simulink model "LOSdemoKF"  (R2016b)
settings: Solver=ode1  StartTime=0.0  StopTime=1200  FixedStep=0.1  RelTol=1e-3
libraries: simulink x1
settings Model: Creator=qys  LastModifiedBy=qys

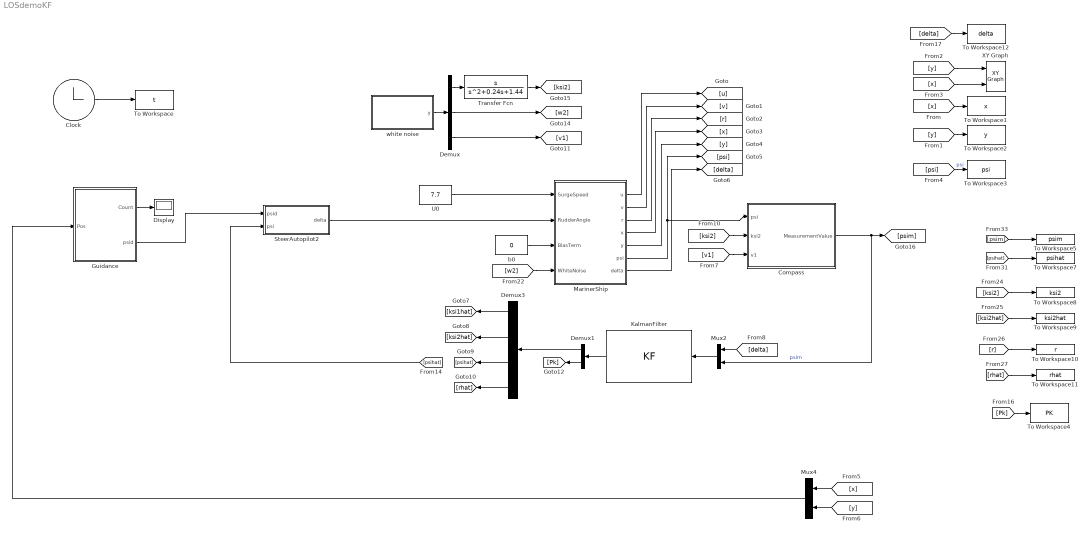
== system LOSdemoKF ==
  Clock : Clock
  Compass : Subsystem
  Demux : Demux  Outputs=3
  Demux1 : Demux  Outputs=[4 16]
  Demux3 : Demux
  Display : Display
  Guidance : Subsystem  mask(Guidance){D=800, R=300, PointSet=[300 300 2900 2500 2900 4800]'}
      mask prompts: D "LookaheadDistance"; R "ChangeRadius"; PointSet "WayPointSet"
      mask help:
      | set lookahead distance\change radius\points number\points set
      | LookaheadDistance: D = 500
      | ChangeRadius: R = 300
      | WayPointSet: PointSet = [0 0 2900 2900 2900 4900 0 0 0 0]'
  KalmanFilter : S-Function  FunctionName=KF  Parameters=Q,R  SFunctionDeploymentMode=off  EnableBusSupport=off  mask(KF4){Q=diag([1e-3 1e-6]), R=1e-2}
      mask prompts: Q "QK"; R "RK"
      mask help:
      | Q = diag([1 1])
      | R = 1
      mask Display: disp('KF4')
  MarinerShip : Subsystem  mask{InitialState=[0;0;0;0;0;0;0]}
      mask Display: disp('mariner1')
  Mux2 : Mux  Inputs=2
  Mux4 : Mux  Inputs=2
  SteerAutopilot2 : Subsystem  mask(PID+TFF){Kp=1.45, Ti=1/100, Td=40}
      mask help:
      | TFF = T*Wxd/K+Wxd/K
      | PID = Kp*[(Xd-X)+Integrate(Xd-X)/Ti+Td*D(Xd-X)]
      | delta = TFF+PID*T/K
      | Kp = T*wn^2/K;
      | Td = T*(2*ksi*wn-1/T)/(K*Kp);
      | Ti = 10/wn;
  To Workspace : ToWorkspace  VariableName=t  SampleTime=-1
  To Workspace1 : ToWorkspace  VariableName=x  SampleTime=-1
  To Workspace10 : ToWorkspace  VariableName=r  SampleTime=-1
  To Workspace11 : ToWorkspace  VariableName=rhat  SampleTime=-1
  To Workspace12 : ToWorkspace  VariableName=delta  SampleTime=-1
  To Workspace2 : ToWorkspace  VariableName=y  SampleTime=-1
  To Workspace3 : ToWorkspace  VariableName=psi  SampleTime=-1
  To Workspace4 : ToWorkspace  VariableName=PK  SampleTime=-1
  To Workspace5 : ToWorkspace  VariableName=psim  SampleTime=-1
  To Workspace7 : ToWorkspace  VariableName=psihat  SampleTime=-1
  To Workspace8 : ToWorkspace  VariableName=ksi2  SampleTime=-1
  To Workspace9 : ToWorkspace  VariableName=ksi2hat  SampleTime=-1
  Transfer Fcn : TransferFcn  Numerator=[1 0]  Denominator=[1 0.24 1.44]
  U0 : Constant  Value=7.7
  XY Graph : simulink/Sinks/XY Graph  xmin=-100  xmax=5000  ymin=-100  ymax=5000  st=-1
  b0 : Constant  Value=0
  white noise : MATLAB Function  TreatAsAtomicUnit=on
  wires:
  U0/1 -> MarinerShip/1(SurgeSpeed)
  Clock/1 -> To Workspace/1
  Mux2/1 -> KalmanFilter/1
  Compass/1(MeasurementValue) -> [psim], Mux2/2  "psim"
  Demux1/1 -> Demux3/1
  Guidance/1(Count) -> Display/1
  Mux4/1 -> Guidance/1(Pos)
  MarinerShip/1(u) -> [u]
  MarinerShip/2(v) -> [v]
  MarinerShip/3(r) -> [r]
  MarinerShip/4(x) -> [x]
  MarinerShip/5(y) -> [y]
  MarinerShip/6(psi) -> [psi], Compass/1(psi)
  MarinerShip/7(delta) -> [delta]
  [x] -> To Workspace1/1
  [y] -> To Workspace2/1
  [y] -> XY Graph/1
  [x] -> XY Graph/2
  [psi] -> To Workspace3/1  "psi"
  Demux3/1 -> [ksi1hat]
  Demux3/2 -> [ksi2hat]
  Demux3/3 -> [psihat]
  Demux3/4 -> [rhat]
  [x] -> Mux4/1
  [y] -> Mux4/2
  Demux1/2 -> [Pk]
  [delta] -> Mux2/1
  [ksi2] -> Compass/2(ksi2)
  [Pk] -> To Workspace4/1
  [psim] -> To Workspace5/1
  [psihat] -> To Workspace7/1
  [ksi2] -> To Workspace8/1
  [ksi2hat] -> To Workspace9/1
  [r] -> To Workspace10/1
  [rhat] -> To Workspace11/1
  [w2] -> MarinerShip/4(WhiteNoise)
  b0/1 -> MarinerShip/3(BiasTerm)
  [delta] -> To Workspace12/1
  Guidance/2(psid) -> SteerAutopilot2/1(psid)
  SteerAutopilot2/1(delta) -> MarinerShip/2(RudderAngle)
  KalmanFilter/1 -> Demux1/1
  [psihat] -> SteerAutopilot2/2(psi)
  Transfer Fcn/1 -> [ksi2]
  white noise/1(y) -> Demux/1
  Demux/1 -> Transfer Fcn/1
  Demux/2 -> [w2]
  Demux/3 -> [v1]
  [v1] -> Compass/3(v1)

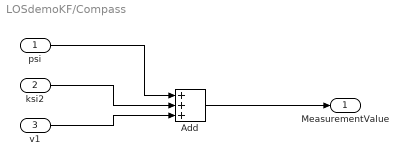
== system LOSdemoKF/Compass ==
  psi : Inport
  ksi2 : Inport  Port=2
  v1 : Inport  Port=3
  Add : Sum  Inputs=+++
  MeasurementValue : Outport
  wires:
  ksi2/1 -> Add/2
  psi/1 -> Add/1
  Add/1 -> MeasurementValue/1
  v1/1 -> Add/3

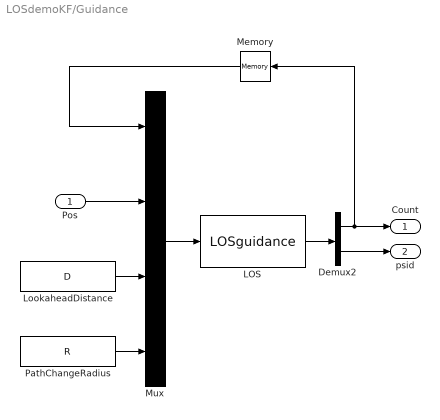
== system LOSdemoKF/Guidance ==
  Pos : Inport
  Demux2 : Demux  Outputs=2
  LOS : S-Function  FunctionName=LOSguidance  Parameters=PointSet  SFunctionDeploymentMode=off  EnableBusSupport=off
  LookaheadDistance : Constant  Value=D
  Memory : Memory  X0=1
  Mux : Mux
  PathChangeRadius : Constant  Value=R
  Count : Outport
  psid : Outport  Port=2
  wires:
  LOS/1 -> Demux2/1
  Demux2/2 -> psid/1
  Pos/1 -> Mux/2
  LookaheadDistance/1 -> Mux/3
  PathChangeRadius/1 -> Mux/4
  Mux/1 -> LOS/1
  Demux2/1 -> Memory/1, Count/1
  Memory/1 -> Mux/1

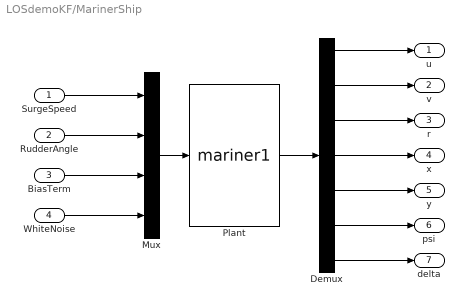
== system LOSdemoKF/MarinerShip ==
  SurgeSpeed : Inport
  RudderAngle : Inport  Port=2
  BiasTerm : Inport  Port=3
  WhiteNoise : Inport  Port=4
  Demux : Demux  Outputs=7
  Mux : Mux
  Plant : S-Function  FunctionName=mariner1  Parameters=InitialState  SFunctionDeploymentMode=off  EnableBusSupport=off
  u : Outport
  v : Outport  Port=2
  r : Outport  Port=3
  x : Outport  Port=4
  y : Outport  Port=5
  psi : Outport  Port=6
  delta : Outport  Port=7
  wires:
  SurgeSpeed/1 -> Mux/1
  RudderAngle/1 -> Mux/2
  BiasTerm/1 -> Mux/3
  WhiteNoise/1 -> Mux/4
  Mux/1 -> Plant/1
  Plant/1 -> Demux/1
  Demux/3 -> r/1
  Demux/4 -> x/1
  Demux/5 -> y/1
  Demux/6 -> psi/1
  Demux/7 -> delta/1
  Demux/2 -> v/1
  Demux/1 -> u/1

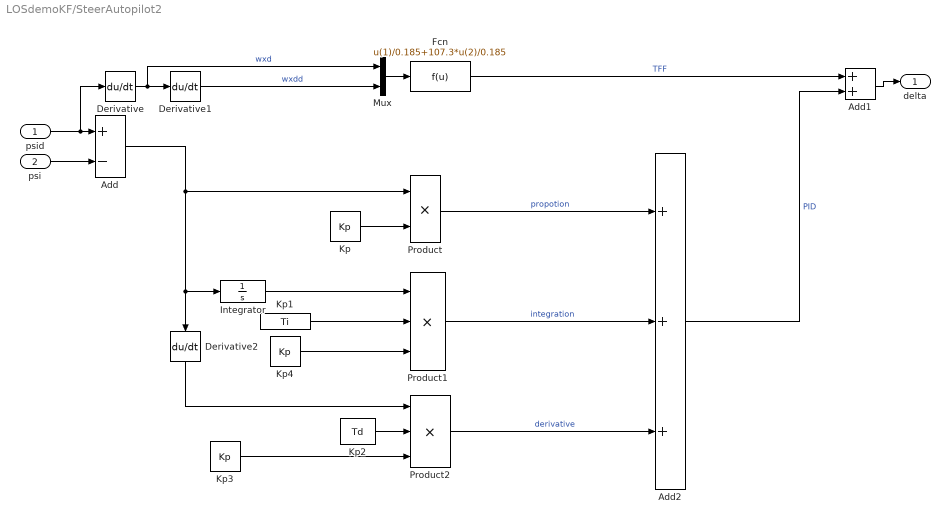
== system LOSdemoKF/SteerAutopilot2 ==
  psid : Inport
  psi : Inport  Port=2
  Add : Sum  Inputs=+-
  Add1 : Sum
  Add2 : Sum  Inputs=+++
  Derivative : Derivative
  Derivative1 : Derivative
  Derivative2 : Derivative
  Fcn : Fcn  Expr=u(1)/0.185+107.3*u(2)/0.185
  Integrator : Integrator
  Kp : Constant  Value=Kp
  Kp1 : Constant  Value=Ti
  Kp2 : Constant  Value=Td
  Kp3 : Constant  Value=Kp
  Kp4 : Constant  Value=Kp
  Mux : Mux  Inputs=2
  Product : Product
  Product1 : Product  Inputs=3
  Product2 : Product  Inputs=3
  delta : Outport
  wires:
  psid/1 -> Derivative/1, Add/1
  psi/1 -> Add/2
  Derivative/1 -> Mux/1, Derivative1/1  "wxd"
  Derivative1/1 -> Mux/2  "wxdd"
  Mux/1 -> Fcn/1
  Fcn/1 -> Add1/1  "TFF"
  Add2/1 -> Add1/2  "PID"
  Add1/1 -> delta/1
  Kp/1 -> Product/2
  Kp1/1 -> Product1/2
  Integrator/1 -> Product1/1
  Derivative2/1 -> Product2/1
  Kp2/1 -> Product2/2
  Product/1 -> Add2/1  "propotion"
  Product1/1 -> Add2/2  "integration"
  Product2/1 -> Add2/3  "derivative"
  Add/1 -> Derivative2/1, Integrator/1, Product/1
  Kp3/1 -> Product2/3
  Kp4/1 -> Product1/3

== matlab function LOSdemoKF/white noise ==
  data: y output
function y = fcn()
Qk = diag([1e-2 1e-20]);
Rk = 1e-1;
w = Qk*randn(2,1);
v = Rk*randn(1,1);
y = [w;v];
